simulink model "test"  (R2022a)
settings: Solver=VariableStepAuto  StartTime=0.0  StopTime=10  RelTol=1e-3
values from neighbouring files (symbols this model uses):
  dt = ds/v    [DefineUAVPath.m]    (also in DronePathPlanSubsystem.m; PathPlanSubsystem.m = ds/speed)
libraries: aerolibanimutils x2
settings Model: Creator=zckog  LastModifiedBy=zckog
settings DebuggingCC: UnconnectedInputMsg=warning  UnconnectedOutputMsg=warning  UnconnectedLineMsg=warning
settings RTWCC: DLArmComputeVersion=19.05

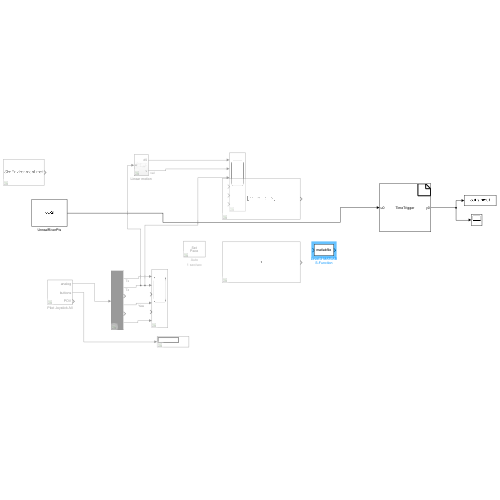
[thumbnail: Simulink's stored preview of the top-level diagram]
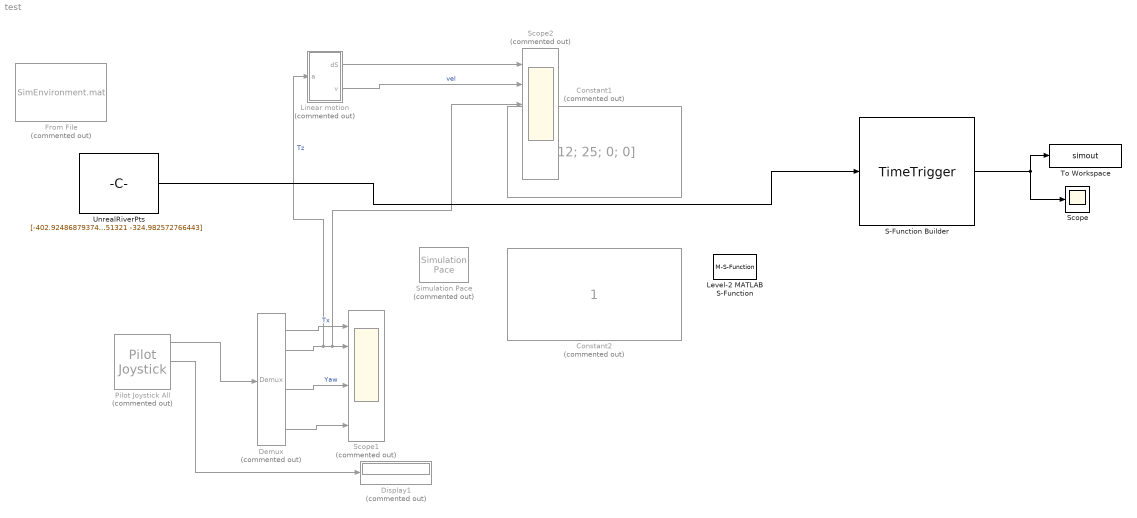
== system test ==
  Constant1 : Constant  Commented=on  Value=[12; 25; 0; 0]  OutDataTypeStr=int32  SampleTime=1
  Constant2 : Constant  Commented=on  OutDataTypeStr=int32  SampleTime=1
  Demux : Demux  Commented=on  Outputs=6
  Display1 : Display  Commented=on
  From File : FromFile  Commented=on  FileName=SimEnvironment.mat  SampleTime=0
  Level-2 MATLAB S-Function : M-S-Function
  Linear motion : Subsystem  Commented=on
  Pilot Joystick All : aerolibanimutils/Pilot Joystick  Commented=on  JoystickID=Joystick1  OutputConfiguration=AllOutputs  SampleTime=dt
  S-Function Builder : S-Function  FunctionName=TimeTrigger  SFunctionModules=TimeTrigger_wrapper  SFunctionDeploymentMode=off  EnableBusSupport=off  mask(S-Function Builder){}
      mask help: Simulink:masks:SFunctionBuilder_MD
      mask init:
      | val = [[.9  0.75 0.75 1 1 .9 .9 1]',[1 1 0.75 0.75 .9 .9 1 .9]'];try , sys = get_param(gcb,'SfunBuilderFcnName');if isempty(sys), sys = get_param(gcb,'FunctionName'); end,catch, sys = get_param(gcb,'FunctionName'); end
      settings: CopyFcn=set_param(gcbh,'LinkStatus','none')  OpenFcn=sfunctionwizard(gcbh)
      mask Display:
      | plot(val(:,1),val(:,2))
      | disp(sys)
      | port_label('input',1,'u0')
      | port_label('output',1,'y0')
  Scope : Scope
  Scope1 : Scope  Commented=on  NumInputPorts=6
  Scope2 : Scope  Commented=on  NumInputPorts=6
  Simulation Pace : aerolibanimutils/Simulation Pace  Commented=on  SimulationPace=1  SleepMode=Auto  OutputPaceError=off  SampleTime=dt
  To Workspace : ToWorkspace  VariableName=simout  SaveFormat=Timeseries  SampleTime=-1
  UnrealRiverPts : Constant  Value=|
      | [-402.924868793743	267.174066483351;
      | -386.279322333391	267.212395336407;
      | -403.147892748961	241.736224883520;
      | -386.323394922344	241.806153769400;
      | -361.163861288494	241.910726171762;
      | -403.284023119093	226.209360117309;
      | -386.350295583676	226.298902747316;
      | -361.027921515931	226.432803093080;
      | -335.798946536105	226.566209560579;
      | -386.368423952853	215.848558498968;
      | -335.598412435239	216.155732951668;
      | -323.806152027249	216.227079816257;
      | -386.391306916241	202.657363939555;
      | -360.820681118613	202.836684988886;
      | -323.489220838432	203.098482126097;
      | -306.587646800272	203.217009064618;
      | -360.633027243144	181.470662410300;
      | -305.926036962295	181.939760692419;
      | -292.317589727332	182.056449605252;
      | -343.489959766660	181.617659776856;
      | -343.104174367082	157.159977802651;
      | -291.424859867265	157.695641610756;
      | -248.656482282387	158.138942227750;
      | -342.754736439567	135.006620754327;
      | -313.160680071436	135.361363466751;
      | -247.470629312756	136.148787349962;
      | -230.288862001445	136.354744474070;
      | -312.539217109257	112.860637741347;
      | -298.532677619770	113.051660676950;
      | -228.929524674218	114.000917173378;
      | -194.394086738495	114.471915790971;
      | -297.677557073314	87.2777352805282;
      | -280.032561641803	87.5517935126713;
      | -192.489112964477	88.9114993212302;
      | -157.786512696434	89.4504925625232;
      | -279.097042160583	64.2282047863231;
      | -266.660809017576	64.4427054747657;
      | -155.749971579296	66.3557004076109;
      | -120.917898166206	66.9564855200379;
      | -265.594022024512	40.7118276866978;
      | -206.739469240256	41.8298450352006;
      | -118.531260962585	43.5054725350186;
      | -74.8571880422759	44.3351172930661;
      | -204.905699903356	14.7340533855086;
      | -151.297164620827	15.8599601810189;
      | -71.6765308595729	17.5321829370069;
      | 7.00839531572296	19.1847536072946;
      | -149.140559197448	-8.59638572525467;
      | -140.165514766095	-8.39156093901602;
      | 10.6006085503716	-4.95083825329373;
      | 19.3640869038875	-4.75084174138847;
      | -135.267819264684	-61.8685092817043;
      | -17.3953962627179	-58.7089888577519;
      | 27.3920574131846	-57.5084801126023;
      | 159.967529781662	-53.9548506715891;
      | -11.7123978061272	-100.660290576105;
      | 60.8805817647659	-98.4851916828967;
      | 168.299670983527	-95.2666002509120;
      | 480.360983260503	-85.9163267264072;
      | 71.6998703556665	-165.213010236890;
      | 500.741735244172	-150.186057611471;
      | 85.9904533276839	-253.349990739424;
      | 142.853773422745	-250.977506020388;
      | 527.613327036968	-234.924342752281;
      | 159.846390086396	-344.351858024191;
      | 556.171941251321	-324.982572766443]
  wires:
  Pilot Joystick All/1 -> Demux/1
  Demux/2 -> Linear motion/1(a), Scope2/3, Scope1/2  "Tz"
  Demux/1 -> Scope1/1  "Tx"
  Demux/4 -> Scope1/4  "Yaw"
  Demux/6 -> Scope1/6
  Pilot Joystick All/2 -> Display1/1
  Linear motion/1(dS) -> Scope2/1
  Linear motion/2(v) -> Scope2/2  "vel"
  S-Function Builder/1 -> To Workspace/1, Scope/1
  UnrealRiverPts/1 -> S-Function Builder/1

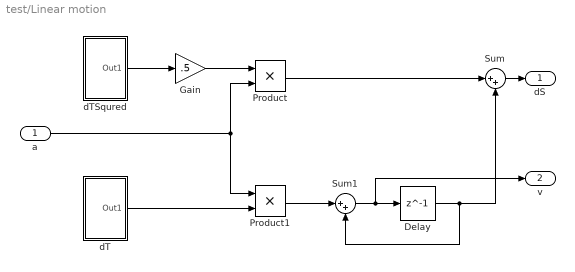
== system test/Linear motion ==
  a : Inport
  Delay : Delay  DelayLength=1  InitialCondition=0
  Gain : Gain  Gain=.5
  Product : Product
  Product1 : Product
  Sum : Sum  Inputs=|++
  Sum1 : Sum  Inputs=|++
  dT : Subsystem
  dTSqured : Subsystem
  dS : Outport
  v : Outport  Port=2
  wires:
  a/1 -> Product/2, Product1/1
  Product1/1 -> Sum1/1
  Delay/1 -> Sum/2, Sum1/2
  dTSqured/1(Out1) -> Gain/1
  Product/1 -> Sum/1
  Gain/1 -> Product/1
  dT/1(Out1) -> Product1/2
  Sum/1 -> dS/1
  Sum1/1 -> v/1, Delay/1

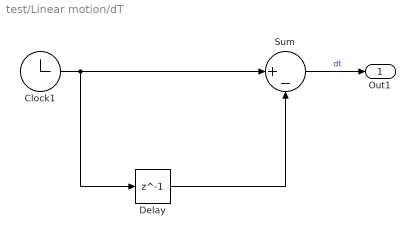
== system test/Linear motion/dT ==
  Clock1 : Clock
  Delay : Delay  DelayLength=1  InitialCondition=0
  Sum : Sum  Inputs=|+-
  Out1 : Outport
  wires:
  Sum/1 -> Out1/1  "dt"
  Clock1/1 -> Sum/1, Delay/1
  Delay/1 -> Sum/2

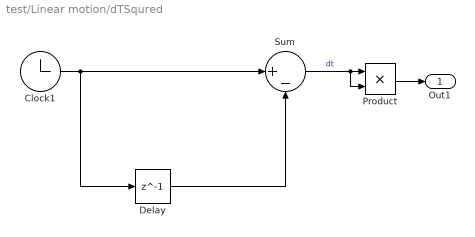
== system test/Linear motion/dTSqured ==
  Clock1 : Clock
  Delay : Delay  DelayLength=1  InitialCondition=0
  Product : Product
  Sum : Sum  Inputs=|+-
  Out1 : Outport
  wires:
  Sum/1 -> Product/2, Product/1  "dt"
  Clock1/1 -> Sum/1, Delay/1
  Delay/1 -> Sum/2
  Product/1 -> Out1/1
